simulink model "snubber_circuit"  (R2019a)
settings: Solver=VariableStepAuto  StartTime=0.0  StopTime=0.5  RelTol=1e-3
libraries: powerlib x5
settings Model: Creator=omer  LastModifiedBy=omer

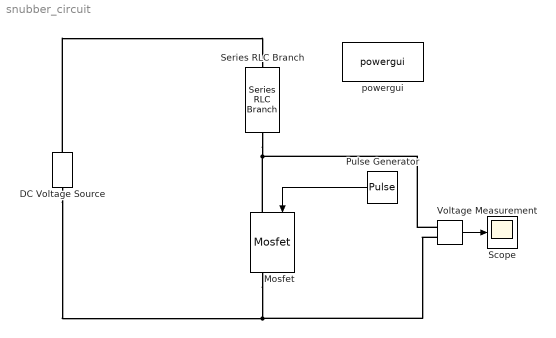
== system snubber_circuit ==
  DC Voltage Source : powerlib/Electrical Sources/DC Voltage Source  Amplitude=36  Measurements=None
      settings: SourceProductName=Simscape Electrical
  Mosfet : powerlib/Power Electronics/Mosfet  Ron=0.032  Lon=0  Rd=0.01  Vfd=1.3  IC=0  Rs=1  Cs=50e-6  Measurements=on
      settings: SourceProductName=Simscape Electrical
  Pulse Generator : DiscretePulseGenerator  PulseType=Time based  Amplitude=10  Period=1/50000  PulseWidth=7.8
  Scope : Scope
  Series RLC Branch : powerlib/Elements/Series RLC Branch  LConnTagsString=__new0  RConnTagsString=__new0  BranchType=RL  Resistance=0.220  Inductance=100e-6  SetiL0=off  InitialCurrent=0.160  Capacitance=1e-6  Setx0=off  InitialVoltage=0  Measurements=None
      settings: SourceProductName=Simscape Electrical
  Voltage Measurement : powerlib/Measurements/Voltage Measurement  PhasorSimulation=off  OutputType=Complex  PSBequivalent=0
      settings: SourceProductName=Simscape Electrical
  powergui : powerlib/powergui  Priority=1  SimulationMode=Continuous  SampleTime=50e-6  frequency=60  Iterations=50  frequencyindice=0  Pbase=100e6  ErrMax=1e-4  UnitsV=kV  UnitsW=MW  buscounter=0  FunctionMessages=off  echomessages=off  EnableUseOfTLC=off  CurrentSourceSwitches=off  DisableSnubberDevices=off  DisableRonSwitches=off  DisableVfSwitches=off  DisplayEquations=off  AutomaticDiscreteSolvers=off  SolverType=Tustin/Backward Euler (TBE)  Interpol=off  ExternalGateDelay=off  methode=off  Ts=100  x0status=blocks  SPID=on  SwTol=0  HookPort=off  NonlinearTolerance=0  nMaxIteration=15  ContinueOnMaxIteration=off  RestoreLinks=warning  ResistiveCurrentMeasurement=off  Frange=[0:2:500]  Ylog=off  Xlog=on  ShowGrid=off  save=off  variable=ZData  structure=0  ZoomFFT=off  StartTime=0.0  cycles=1  DisplayStyle=1  fundamental=60  FreqAxis=off  MaxFrequency=1000  frequencyindicesteady=1  RmsSteady=1  display=off
      settings: SourceProductName=Simscape Electrical
  wires:
  Pulse Generator/1 -> Mosfet/1
  Voltage Measurement/1 -> Scope/1
  connections:
  DC Voltage Source/RConn1 -- Series RLC Branch/LConn1
  DC Voltage Source/LConn1 -- Mosfet/RConn1 -- Voltage Measurement/LConn2
  Series RLC Branch/RConn1 -- Mosfet/LConn1 -- Voltage Measurement/LConn1
